simulink model "TireModel"  (R2026b)
settings: Solver=ode45  StopTime=1
settings Model: DataDictionary=VehicleData.sldd  Creator=Xu Dingyi  LastModifiedBy=29358

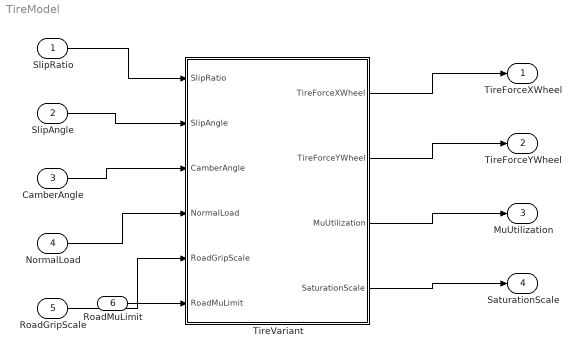
== system TireModel ==
  SlipRatio : Inport  PortDimensions=4
  SlipAngle : Inport  Port=2  PortDimensions=4
  CamberAngle : Inport  Port=3  PortDimensions=4
  NormalLoad : Inport  Port=4  PortDimensions=4
  RoadGripScale : Inport  Port=5  PortDimensions=4
  RoadMuLimit : Inport  Port=6  PortDimensions=4
  TireVariant : Subsystem  Variant=on
  TireForceXWheel : Outport
  TireForceYWheel : Outport  Port=2
  MuUtilization : Outport  Port=3
  SaturationScale : Outport  Port=4
  wires:
  SlipRatio/1 -> TireVariant/1(SlipRatio)
  SlipAngle/1 -> TireVariant/2(SlipAngle)
  CamberAngle/1 -> TireVariant/3(CamberAngle)
  NormalLoad/1 -> TireVariant/4(NormalLoad)
  RoadGripScale/1 -> TireVariant/5(RoadGripScale)
  TireVariant/1(TireForceXWheel) -> TireForceXWheel/1
  TireVariant/2(TireForceYWheel) -> TireForceYWheel/1
  TireVariant/3(MuUtilization) -> MuUtilization/1
  TireVariant/4(SaturationScale) -> SaturationScale/1
  RoadMuLimit/1 -> TireVariant/6(RoadMuLimit)

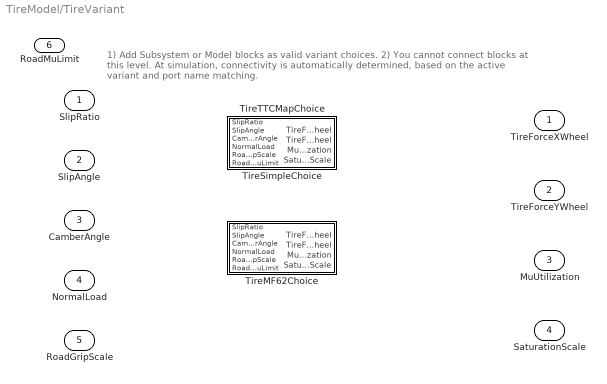
== system TireModel/TireVariant ==
  note: 1) Add Subsystem or Model blocks as valid variant choices.
      | 2) You cannot connect blocks at this level. At simulation, connectivity is automatically
      | determined, based on the active variant and port name matching.
  SlipRatio : Inport  PortDimensions=4
  SlipAngle : Inport  Port=2  PortDimensions=4
  CamberAngle : Inport  Port=3  PortDimensions=4
  NormalLoad : Inport  Port=4  PortDimensions=4
  RoadGripScale : Inport  Port=5  PortDimensions=4
  RoadMuLimit : Inport  Port=6  PortDimensions=4
  TireMF62Choice : Subsystem  VariantControl=TireSelection.ModelMode == 1
  TireSimpleChoice : Subsystem  VariantControl=TireSelection.ModelMode == 0
  TireTTCMapChoice : Subsystem  VariantControl=TireSelection.ModelMode == 2
  TireForceXWheel : Outport
  TireForceYWheel : Outport  Port=2
  MuUtilization : Outport  Port=3
  SaturationScale : Outport  Port=4

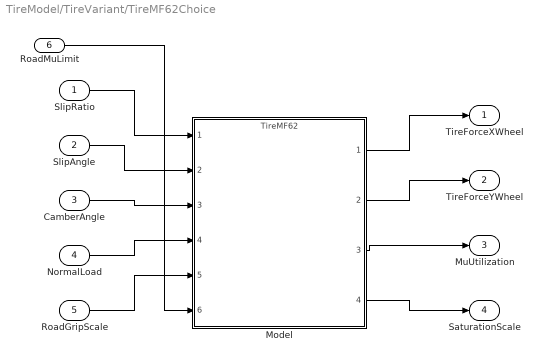
== system TireModel/TireVariant/TireMF62Choice ==
  SlipRatio : Inport  PortDimensions=4
  SlipAngle : Inport  Port=2  PortDimensions=4
  CamberAngle : Inport  Port=3  PortDimensions=4
  NormalLoad : Inport  Port=4  PortDimensions=4
  RoadGripScale : Inport  Port=5  PortDimensions=4
  RoadMuLimit : Inport  Port=6  PortDimensions=4
  Model : ModelReference  ModelNameDialog=TireMF62  SimulationMode=Normal  ModelReferenceVersion=2.0
  TireForceXWheel : Outport
  TireForceYWheel : Outport  Port=2
  MuUtilization : Outport  Port=3
  SaturationScale : Outport  Port=4
  wires:
  SlipRatio/1 -> Model/1
  SlipAngle/1 -> Model/2
  CamberAngle/1 -> Model/3
  NormalLoad/1 -> Model/4
  RoadGripScale/1 -> Model/5
  Model/1 -> TireForceXWheel/1
  Model/2 -> TireForceYWheel/1
  Model/3 -> MuUtilization/1
  Model/4 -> SaturationScale/1
  RoadMuLimit/1 -> Model/6

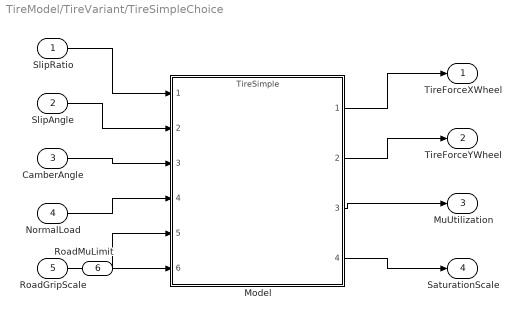
== system TireModel/TireVariant/TireSimpleChoice ==
  SlipRatio : Inport  PortDimensions=4
  SlipAngle : Inport  Port=2  PortDimensions=4
  CamberAngle : Inport  Port=3  PortDimensions=4
  NormalLoad : Inport  Port=4  PortDimensions=4
  RoadGripScale : Inport  Port=5  PortDimensions=4
  RoadMuLimit : Inport  Port=6  PortDimensions=4
  Model : ModelReference  ModelNameDialog=TireSimple  SimulationMode=Normal  ModelReferenceVersion=1.7
  TireForceXWheel : Outport
  TireForceYWheel : Outport  Port=2
  MuUtilization : Outport  Port=3
  SaturationScale : Outport  Port=4
  wires:
  SlipRatio/1 -> Model/1
  SlipAngle/1 -> Model/2
  CamberAngle/1 -> Model/3
  NormalLoad/1 -> Model/4
  RoadGripScale/1 -> Model/5
  Model/1 -> TireForceXWheel/1
  Model/2 -> TireForceYWheel/1
  Model/3 -> MuUtilization/1
  Model/4 -> SaturationScale/1
  RoadMuLimit/1 -> Model/6

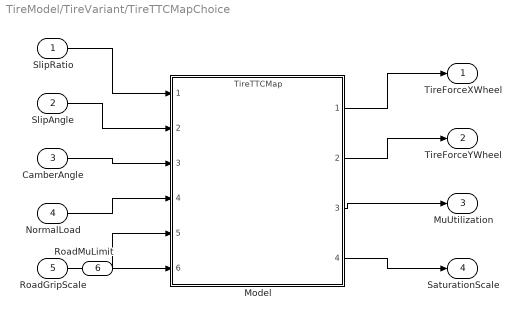
== system TireModel/TireVariant/TireTTCMapChoice ==
  SlipRatio : Inport  PortDimensions=4
  SlipAngle : Inport  Port=2  PortDimensions=4
  CamberAngle : Inport  Port=3  PortDimensions=4
  NormalLoad : Inport  Port=4  PortDimensions=4
  RoadGripScale : Inport  Port=5  PortDimensions=4
  RoadMuLimit : Inport  Port=6  PortDimensions=4
  Model : ModelReference  ModelNameDialog=TireTTCMap  SimulationMode=Normal  ModelReferenceVersion=1.2
  TireForceXWheel : Outport
  TireForceYWheel : Outport  Port=2
  MuUtilization : Outport  Port=3
  SaturationScale : Outport  Port=4
  wires:
  SlipRatio/1 -> Model/1
  SlipAngle/1 -> Model/2
  CamberAngle/1 -> Model/3
  NormalLoad/1 -> Model/4
  RoadGripScale/1 -> Model/5
  Model/1 -> TireForceXWheel/1
  Model/2 -> TireForceYWheel/1
  Model/3 -> MuUtilization/1
  Model/4 -> SaturationScale/1
  RoadMuLimit/1 -> Model/6
